simulink model "Adaptive_safe"  (R2018b)
settings: Solver=VariableStepAuto  StartTime=0.0  StopTime=60  RelTol=1e-3
libraries: simulink x2, Solver_SF x1
settings Model: Creator=周迅  LastModifiedBy=周迅

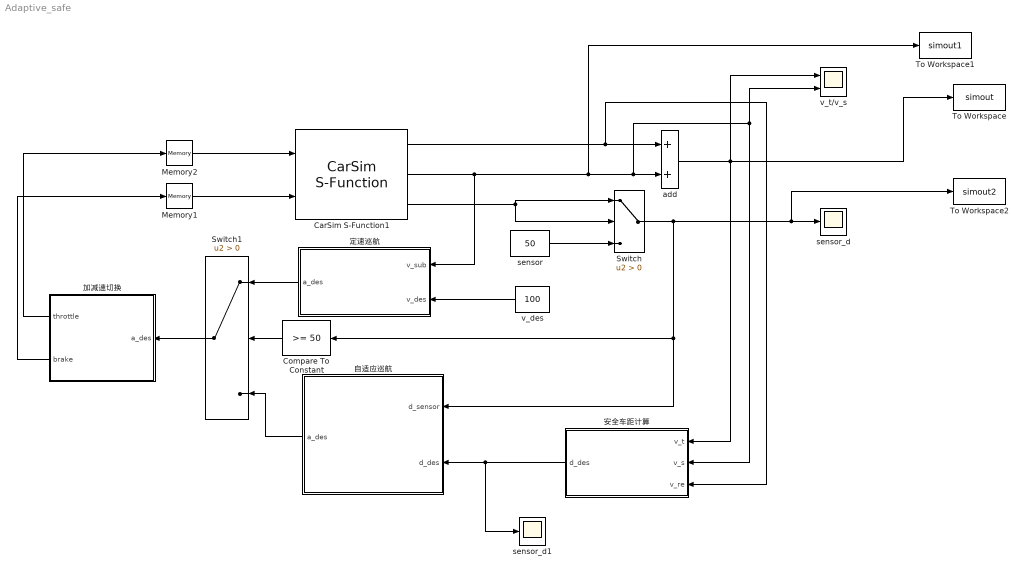
== system Adaptive_safe ==
  CarSim S-Function1 : Solver_SF/CarSim S-Function  Priority=1  SIMFILE=Simfile.sim
  Compare To Constant : simulink/Logic and Bit Operations/Compare To Constant  relop=>=  const=50  OutDataTypeStr=boolean
  Memory1 : Memory
  Memory2 : Memory
  Switch : Switch  Criteria=u2 > Threshold
  Switch1 : Switch  Criteria=u2 > Threshold
  To Workspace : ToWorkspace  VariableName=simout  SaveFormat=Timeseries  SampleTime=-1
  To Workspace1 : ToWorkspace  VariableName=simout1  SaveFormat=Timeseries  SampleTime=-1
  To Workspace2 : ToWorkspace  VariableName=simout2  SaveFormat=Timeseries  SampleTime=-1
  add : Sum
  "sensor " : Constant  Value=50
  sensor_d : Scope
  sensor_d1 : Scope
  v_des : Constant  Value=100
  v_t/v_s : Scope  NumInputPorts=2
  加减速切换 : Subsystem
  安全车距计算 : Subsystem
  定速巡航 : Subsystem
  自适应巡航 : Subsystem
  wires:
  Switch/1 -> To Workspace2/1, sensor_d/1, Compare To Constant/1, 自适应巡航/1(d_sensor)
  Compare To Constant/1 -> Switch1/2
  "sensor "/1 -> Switch/3
  自适应巡航/1(a_des) -> Switch1/3
  v_des/1 -> 定速巡航/2(v_des)
  CarSim S-Function1/3 -> Switch/1, Switch/2
  CarSim S-Function1/1 -> add/1, 安全车距计算/3(v_re)
  Switch1/1 -> 加减速切换/1(a_des)
  加减速切换/2(brake) -> Memory1/1
  CarSim S-Function1/2 -> 定速巡航/1(v_sub), To Workspace1/1, 安全车距计算/2(v_s), v_t/v_s/2, add/2
  add/1 -> To Workspace/1, 安全车距计算/1(v_t), v_t/v_s/1
  定速巡航/1(a_des) -> Switch1/1
  安全车距计算/1(d_des) -> sensor_d1/1, 自适应巡航/2("d_des ")
  Memory1/1 -> CarSim S-Function1/2
  加减速切换/1(throttle) -> Memory2/1
  Memory2/1 -> CarSim S-Function1/1

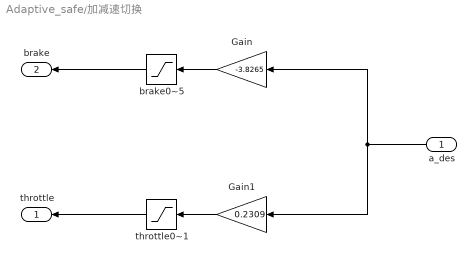
== system Adaptive_safe/加减速切换 ==
  a_des : Inport
  Gain : Gain  Gain=-3.8265
  Gain1 : Gain  Gain=0.2309
  brake0~5 : Saturate  UpperLimit=10  LowerLimit=0
  throttle0~1 : Saturate  UpperLimit=1  LowerLimit=0
  throttle : Outport
  brake : Outport  Port=2
  wires:
  a_des/1 -> Gain/1, Gain1/1
  Gain1/1 -> throttle0~1/1
  Gain/1 -> brake0~5/1
  throttle0~1/1 -> throttle/1
  brake0~5/1 -> brake/1

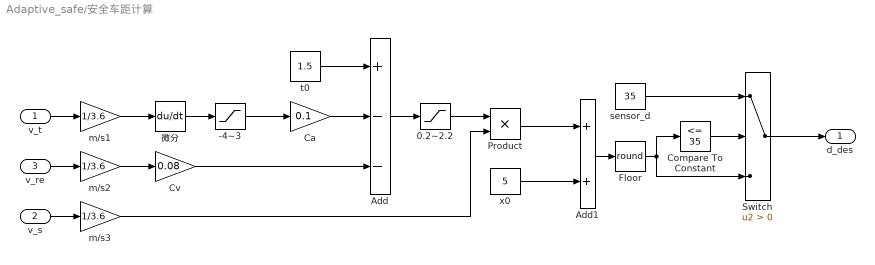
== system Adaptive_safe/安全车距计算 ==
  v_t : Inport
  v_s : Inport  Port=2
  v_re : Inport  Port=3
  -4~3 : Saturate  UpperLimit=3  LowerLimit=-4
  0.2~2.2 : Saturate  UpperLimit=2.2  LowerLimit=0.2
  Add : Sum  Inputs=+--
  Add1 : Sum
  Ca : Gain  Gain=0.1
  Compare To Constant : simulink/Logic and Bit Operations/Compare To Constant  relop=<=  const=35  OutDataTypeStr=boolean
  Cv : Gain  Gain=0.08
  Floor : Rounding  Operator=round
  Product : Product
  Switch : Switch  Criteria=u2 > Threshold
  m/s1 : Gain  Gain=1/3.6
  m/s2 : Gain  Gain=1/3.6
  m/s3 : Gain  Gain=1/3.6
  sensor_d : Constant  Value=35
  t0 : Constant  Value=1.5
  x0 : Constant  Value=5
  微分 : Derivative
  d_des : Outport
  wires:
  Add/1 -> 0.2~2.2/1
  v_s/1 -> m/s3/1
  v_t/1 -> m/s1/1
  t0/1 -> Add/1
  Add1/1 -> Floor/1
  Product/1 -> Add1/1
  x0/1 -> Add1/2
  v_re/1 -> m/s2/1
  Cv/1 -> Add/3
  微分/1 -> -4~3/1
  Ca/1 -> Add/2
  -4~3/1 -> Ca/1
  m/s1/1 -> 微分/1
  m/s2/1 -> Cv/1
  m/s3/1 -> Product/2
  Compare To Constant/1 -> Switch/2
  sensor_d/1 -> Switch/1
  Floor/1 -> Switch/3, Compare To Constant/1
  0.2~2.2/1 -> Product/1
  Switch/1 -> d_des/1

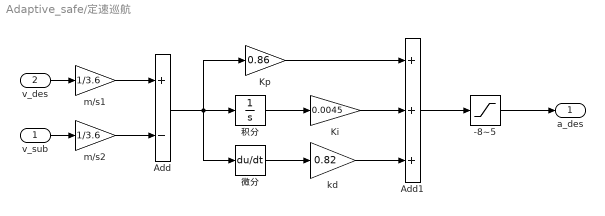
== system Adaptive_safe/定速巡航 ==
  v_sub : Inport
  v_des : Inport  Port=2
  -8~5 : Saturate  UpperLimit=5  LowerLimit=-5
  Add : Sum  Inputs=+-
  Add1 : Sum  Inputs=+++
  Ki : Gain  Gain=0.0045
  Kp : Gain  Gain=0.86
  kd : Gain  Gain=0.82
  m/s1 : Gain  Gain=1/3.6
  m/s2 : Gain  Gain=1/3.6
  微分 : Derivative
  积分 : Integrator
  a_des : Outport
  wires:
  Add/1 -> 积分/1, 微分/1, Kp/1
  积分/1 -> Ki/1
  Ki/1 -> Add1/2
  微分/1 -> kd/1
  kd/1 -> Add1/3
  Kp/1 -> Add1/1
  v_des/1 -> m/s1/1
  v_sub/1 -> m/s2/1
  Add1/1 -> -8~5/1
  -8~5/1 -> a_des/1
  m/s1/1 -> Add/1
  m/s2/1 -> Add/2

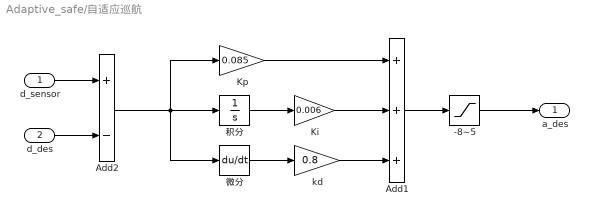
== system Adaptive_safe/自适应巡航 ==
  d_sensor : Inport
  "d_des " : Inport  Port=2
  -8~5 : Saturate  UpperLimit=5  LowerLimit=-5
  Add1 : Sum  Inputs=+++
  Add2 : Sum  Inputs=+-
  Ki : Gain  Gain=0.006
  Kp : Gain  Gain=0.085
  kd : Gain  Gain=0.8
  微分 : Derivative
  积分 : Integrator
  a_des : Outport
  wires:
  积分/1 -> Ki/1
  Ki/1 -> Add1/2
  微分/1 -> kd/1
  kd/1 -> Add1/3
  Kp/1 -> Add1/1
  Add1/1 -> -8~5/1
  -8~5/1 -> a_des/1
  Add2/1 -> 微分/1, Kp/1, 积分/1
  d_sensor/1 -> Add2/1
  "d_des "/1 -> Add2/2
